simulink model "k1modalbs"  (Simulink 8.6)
settings: Solver=VariableStepAuto  StartTime=0.0  StopTime=10.0  RelTol=1e-3
libraries: cdsIPCx x16, cdsAdcx0 x1, VISMODAL_MASTER x1, cdsParameters x1
settings Model: Creator=controls  LastModifiedBy=controls
settings DataIOCC: SaveFormat=Dataset  SignalLoggingSaveFormat=Dataset
settings OptimizationCC: ExpressionDepthLimit=128
settings DebuggingCC: UnderspecifiedInitializationDetection=Simplified  MergeDetectMultiDrivingBlocksExec=error  SolverPrmCheckMsg=none  FcnCallInpInsideContextMsg=EnableAllAsError  StateNameClashWarn=none
settings HardwareCC: ProdBitPerPointer=64  ProdLargestAtomicFloat=Float  ProdIntDivRoundTo=Zero  ProdEndianess=LittleEndian  ProdWordSize=64  ProdHWDeviceType=Intel->x86-64 (Windows64)
settings GRTTargetCC: GeneratePreprocessorConditionals=Use local settings  CombineOutputUpdateFcns=on  GRTInterface=off
settings ConfigComp: CovModelRefEnable=off

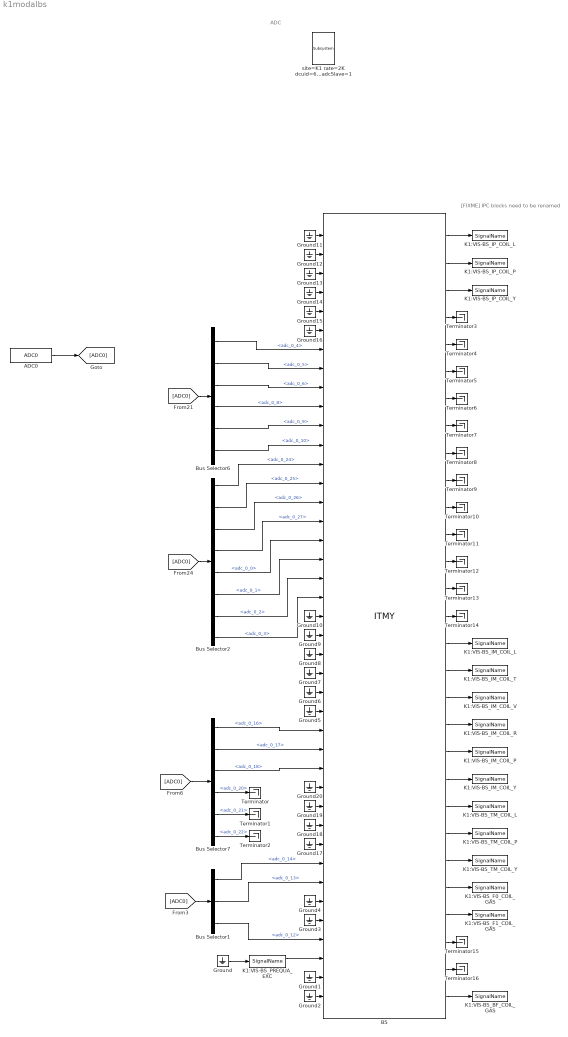
== system k1modalbs ==
  note: ADC
  note: [FIXME] IPC blocks need to be renamed
  ADC0 : cdsAdcx0/ADC0  Tag=cdsAdc  Description=|
      | type-GSC_16AI64SSA
      | card_num=0
      settings: AttributesFormatString=%<Description>\n%<Tag>
  BS : VISMODAL_MASTER/ITMY
  Bus Selector1 : BusSelector  Description=ADC Selector  OutputSignals=adc_0_14,adc_0_13,adc_0_12
      settings: AttributesFormatString=%<Description>
  Bus Selector2 : BusSelector  Description=ADC Selector  OutputSignals=adc_0_24,adc_0_25,adc_0_26,adc_0_27,adc_0_0,adc_0_1,adc_0_2,adc_0_3
      settings: AttributesFormatString=%<Description>
  Bus Selector6 : BusSelector  Description=ADC Selector  OutputSignals=adc_0_4,adc_0_5,adc_0_6,adc_0_8,adc_0_9,adc_0_10
      settings: AttributesFormatString=%<Description>
  Bus Selector7 : BusSelector  Description=ADC Selector  OutputSignals=adc_0_16,adc_0_17,adc_0_18,adc_0_20,adc_0_21,adc_0_22
      settings: AttributesFormatString=%<Description>
  Ground{,1..20} (21 alike) : Ground
  K1:VIS-BS_BF_COIL_GAS : cdsIPCx/SignalName  Tag=cdsIPCx_SHMEM  Description=Inter-Process Communication via Shared memory.
      settings: AttributesFormatString=%<Tag>
  K1:VIS-BS_F0_COIL_GAS : cdsIPCx/SignalName  Tag=cdsIPCx_SHMEM  Description=Inter-Process Communication via Shared memory.
      settings: AttributesFormatString=%<Tag>
  K1:VIS-BS_F1_COIL_GAS : cdsIPCx/SignalName  Tag=cdsIPCx_SHMEM  Description=Inter-Process Communication via Shared memory.
      settings: AttributesFormatString=%<Tag>
  K1:VIS-BS_IM_COIL_L : cdsIPCx/SignalName  Tag=cdsIPCx_SHMEM  Description=Inter-Process Communication via Shared memory.
      settings: AttributesFormatString=%<Tag>
  K1:VIS-BS_IM_COIL_P : cdsIPCx/SignalName  Tag=cdsIPCx_SHMEM  Description=Inter-Process Communication via Shared memory.
      settings: AttributesFormatString=%<Tag>
  K1:VIS-BS_IM_COIL_R : cdsIPCx/SignalName  Tag=cdsIPCx_SHMEM  Description=Inter-Process Communication via Shared memory.
      settings: AttributesFormatString=%<Tag>
  K1:VIS-BS_IM_COIL_T : cdsIPCx/SignalName  Tag=cdsIPCx_SHMEM  Description=Inter-Process Communication via Shared memory.
      settings: AttributesFormatString=%<Tag>
  K1:VIS-BS_IM_COIL_V : cdsIPCx/SignalName  Tag=cdsIPCx_SHMEM  Description=Inter-Process Communication via Shared memory.
      settings: AttributesFormatString=%<Tag>
  K1:VIS-BS_IM_COIL_Y : cdsIPCx/SignalName  Tag=cdsIPCx_SHMEM  Description=Inter-Process Communication via Shared memory.
      settings: AttributesFormatString=%<Tag>
  K1:VIS-BS_IP_COIL_L : cdsIPCx/SignalName  Tag=cdsIPCx_SHMEM  Description=Inter-Process Communication via Shared memory.
      settings: AttributesFormatString=%<Tag>
  K1:VIS-BS_IP_COIL_P : cdsIPCx/SignalName  Tag=cdsIPCx_SHMEM  Description=Inter-Process Communication via Shared memory.
      settings: AttributesFormatString=%<Tag>
  K1:VIS-BS_IP_COIL_Y : cdsIPCx/SignalName  Tag=cdsIPCx_SHMEM  Description=Inter-Process Communication via Shared memory.
      settings: AttributesFormatString=%<Tag>
  K1:VIS-BS_PREQUA_EXC : cdsIPCx/SignalName  Tag=cdsIPCx_SHMEM  Description=Inter-Process Communication via Shared memory.
      settings: AttributesFormatString=%<Tag>
  K1:VIS-BS_TM_COIL_L : cdsIPCx/SignalName  Tag=cdsIPCx_SHMEM  Description=Inter-Process Communication via Shared memory.
      settings: AttributesFormatString=%<Tag>
  K1:VIS-BS_TM_COIL_P : cdsIPCx/SignalName  Tag=cdsIPCx_SHMEM  Description=Inter-Process Communication via Shared memory.
      settings: AttributesFormatString=%<Tag>
  K1:VIS-BS_TM_COIL_Y : cdsIPCx/SignalName  Tag=cdsIPCx_SHMEM  Description=Inter-Process Communication via Shared memory.
      settings: AttributesFormatString=%<Tag>
  Terminator{,1..16} (17 alike) : Terminator
  site=K1 rate=2K dcuid=62 host=k1bs specific_cpu=4 adcSlave=1 : cdsParameters/Subsystem  Tag=cdsParameters  Description=|
      | Purpose:                                                                                                                                                                                                                                
      | Provide system parameters to the FE code generator to properly configure the generated EPICS names, rep rate of the FE controller, and the Data Acquisition node ID for proper storage of data from this FE controller.                 
      |                                                                                                                                                                                                                                         
      | Useage:                                                                                                                                                                                                                                 
      | The part NAME field is used to identify the FE parameters. It must be of the form:                                                                                                                                                      
      | site=                                                                                                                                                                                                                                   
      | rate=                                                                                                                                                                                                                                   
      | dcuid=                                                                                                                                                                                                                                  
      |                                                                                                                                                                                                                                         
      | Where:                                                                                                                                                                                                                                  
      | site= argument may be H1, H2, L1, M1, G1, either as a single argument or multiple, for example site=H1,H2. These are the only names allowed. These will become the first two characters of all EPICS and signal names (for example G1:).
      |                                                                                                                                                                                                                                         
      | rate= may be 2K, 16K, 32K, or 64K                                                                                                                                                                                                       
      |                                                                                                                                                                                                                                         
      | dcuid= is site specific ie it must be unique at each site.
      settings: AttributesFormatString=%<Tag>
  wires:
  BS/16 -> K1:VIS-BS_IM_COIL_L/1
  BS/17 -> K1:VIS-BS_IM_COIL_T/1
  BS/18 -> K1:VIS-BS_IM_COIL_V/1
  BS/19 -> K1:VIS-BS_IM_COIL_R/1
  BS/20 -> K1:VIS-BS_IM_COIL_P/1
  BS/21 -> K1:VIS-BS_IM_COIL_Y/1
  BS/22 -> K1:VIS-BS_TM_COIL_L/1
  BS/23 -> K1:VIS-BS_TM_COIL_P/1
  BS/24 -> K1:VIS-BS_TM_COIL_Y/1
  BS/1 -> K1:VIS-BS_IP_COIL_L/1
  BS/2 -> K1:VIS-BS_IP_COIL_P/1
  BS/3 -> K1:VIS-BS_IP_COIL_Y/1
  BS/25 -> K1:VIS-BS_F0_COIL_GAS/1
  BS/26 -> K1:VIS-BS_F1_COIL_GAS/1
  BS/29 -> K1:VIS-BS_BF_COIL_GAS/1
  K1:VIS-BS_PREQUA_EXC/1 -> BS/39
  Ground/1 -> K1:VIS-BS_PREQUA_EXC/1
  Ground1/1 -> BS/40
  Ground2/1 -> BS/41
  ADC0/1 -> [ADC0]
  [ADC0] -> Bus Selector6/1
  Bus Selector6/1 -> BS/7  "<adc_0_4>"
  Bus Selector6/2 -> BS/8  "<adc_0_5>"
  Bus Selector6/3 -> BS/9  "<adc_0_6>"
  Bus Selector6/4 -> BS/10  "<adc_0_8>"
  Bus Selector6/5 -> BS/11  "<adc_0_9>"
  Bus Selector6/6 -> BS/12  "<adc_0_10>"
  [ADC0] -> Bus Selector2/1
  Bus Selector2/1 -> BS/13  "<adc_0_24>"
  Bus Selector2/2 -> BS/14  "<adc_0_25>"
  Bus Selector2/3 -> BS/15  "<adc_0_26>"
  Bus Selector2/4 -> BS/16  "<adc_0_27>"
  Bus Selector2/5 -> BS/17  "<adc_0_0>"
  Bus Selector2/6 -> BS/18  "<adc_0_1>"
  Bus Selector2/7 -> BS/19  "<adc_0_2>"
  Bus Selector2/8 -> BS/20  "<adc_0_3>"
  [ADC0] -> Bus Selector7/1
  [ADC0] -> Bus Selector1/1
  Bus Selector1/2 -> BS/35  "<adc_0_13>"
  Bus Selector1/3 -> BS/38  "<adc_0_12>"
  Bus Selector7/1 -> BS/27  "<adc_0_16>"
  Bus Selector7/3 -> BS/29  "<adc_0_18>"
  Bus Selector1/1 -> BS/34  "<adc_0_14>"
  Bus Selector7/2 -> BS/28  "<adc_0_17>"
  Bus Selector7/4 -> Terminator/1  "<adc_0_20>"
  Bus Selector7/6 -> Terminator2/1  "<adc_0_22>"
  Bus Selector7/5 -> Terminator1/1  "<adc_0_21>"
  Ground3/1 -> BS/37
  Ground4/1 -> BS/36
  Ground5/1 -> BS/26
  Ground6/1 -> BS/25
  Ground7/1 -> BS/24
  Ground8/1 -> BS/23
  Ground9/1 -> BS/22
  Ground10/1 -> BS/21
  Ground11/1 -> BS/1
  Ground12/1 -> BS/2
  Ground13/1 -> BS/3
  Ground14/1 -> BS/4
  Ground15/1 -> BS/5
  Ground16/1 -> BS/6
  Ground17/1 -> BS/33
  Ground18/1 -> BS/32
  Ground19/1 -> BS/31
  Ground20/1 -> BS/30
  BS/4 -> Terminator3/1
  BS/5 -> Terminator4/1
  BS/6 -> Terminator5/1
  BS/7 -> Terminator6/1
  BS/8 -> Terminator7/1
  BS/9 -> Terminator8/1
  BS/10 -> Terminator9/1
  BS/11 -> Terminator10/1
  BS/12 -> Terminator11/1
  BS/13 -> Terminator12/1
  BS/14 -> Terminator13/1
  BS/15 -> Terminator14/1
  BS/27 -> Terminator15/1
  BS/28 -> Terminator16/1
